simulink model "newStateflow"  (R2018a)
settings: Solver=VariableStepAuto  StartTime=0.0  StopTime=inf  RelTol=1e-3
settings Model: Creator=alex  LastModifiedBy=rohan

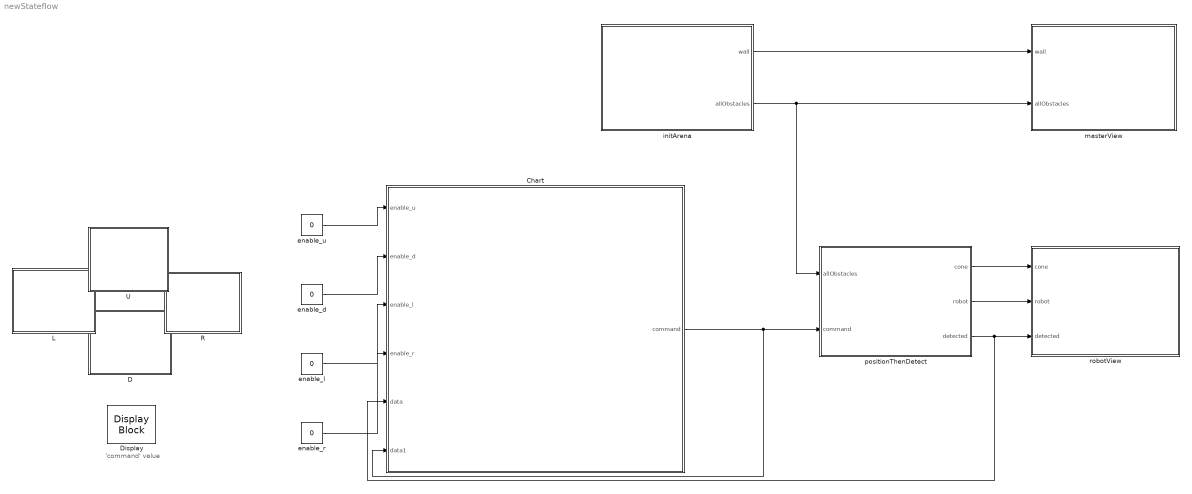
== system newStateflow ==
  note: 'command' value
  Chart : Stateflow chart  TreatAsAtomicUnit=on
  D : Subsystem  DialogController=hmiCreateDDGDialog  IsWebBlock=on  mask(MWDashboardBlock){webBlockId=1a5e94ef-030e-49cd-b944-b929b04abc70, webBlockType=pushbutton, ShowInLibBrwoser=on, ShowInitialText=on, HMISrcModelName=noCollision}
      mask prompts: webBlockId "WebBlock Id"; webBlockType "WebBlock Type"; HMISrcModelName "Source Model"
      mask help: SimulinkHMI:dialogs:PushButtonDialogDesc
      mask Help: helpview([docroot '/mapfiles/simulink.map'], 'hmi_push_button')
      mask Display:
      | model = bdroot(gcb);
      | if strcmp(get_param(model,'BlockDiagramType'), 'library')
      |     image([(matlabroot) '/toolbox/simulink/hmi/icons/PushButton.png']);
      | end
  Display : DisplayBlock  WebBlockId=14  LabelPosition=Hide
  "L " : Subsystem  DialogController=hmiCreateDDGDialog  IsWebBlock=on  mask(MWDashboardBlock){webBlockId=f6d6ee6b-2047-45ee-ab2e-570b521bf019, webBlockType=pushbutton, ShowInLibBrwoser=on, ShowInitialText=on, HMISrcModelName=noCollision}
      mask prompts: webBlockId "WebBlock Id"; webBlockType "WebBlock Type"; HMISrcModelName "Source Model"
      mask help: SimulinkHMI:dialogs:PushButtonDialogDesc
      mask Help: helpview([docroot '/mapfiles/simulink.map'], 'hmi_push_button')
      mask Display:
      | model = bdroot(gcb);
      | if strcmp(get_param(model,'BlockDiagramType'), 'library')
      |     image([(matlabroot) '/toolbox/simulink/hmi/icons/PushButton.png']);
      | end
  R : Subsystem  DialogController=hmiCreateDDGDialog  IsWebBlock=on  mask(MWDashboardBlock){webBlockId=5b3cd59d-fae2-469c-adcb-5a1af564bf62, webBlockType=pushbutton, ShowInLibBrwoser=on, ShowInitialText=on, HMISrcModelName=noCollision}
      mask prompts: webBlockId "WebBlock Id"; webBlockType "WebBlock Type"; HMISrcModelName "Source Model"
      mask help: SimulinkHMI:dialogs:PushButtonDialogDesc
      mask Help: helpview([docroot '/mapfiles/simulink.map'], 'hmi_push_button')
      mask Display:
      | model = bdroot(gcb);
      | if strcmp(get_param(model,'BlockDiagramType'), 'library')
      |     image([(matlabroot) '/toolbox/simulink/hmi/icons/PushButton.png']);
      | end
  U : Subsystem  DialogController=hmiCreateDDGDialog  IsWebBlock=on  mask(MWDashboardBlock){webBlockId=418d2ee9-92ed-471b-995b-1589f387356b, webBlockType=pushbutton, ShowInLibBrwoser=on, ShowInitialText=on, HMISrcModelName=noCollision}
      mask prompts: webBlockId "WebBlock Id"; webBlockType "WebBlock Type"; HMISrcModelName "Source Model"
      mask help: SimulinkHMI:dialogs:PushButtonDialogDesc
      mask Help: helpview([docroot '/mapfiles/simulink.map'], 'hmi_push_button')
      mask Display:
      | model = bdroot(gcb);
      | if strcmp(get_param(model,'BlockDiagramType'), 'library')
      |     image([(matlabroot) '/toolbox/simulink/hmi/icons/PushButton.png']);
      | end
  "enable_d " : Constant  Value=0
  "enable_l " : Constant  Value=0
  "enable_r " : Constant  Value=0
  "enable_u " : Constant  Value=0
  initArena : MATLAB Function  TreatAsAtomicUnit=on
  masterView : MATLAB Function  TreatAsAtomicUnit=on
  positionThenDetect : MATLAB Function  TreatAsAtomicUnit=on
  robotView : MATLAB Function  TreatAsAtomicUnit=on
  wires:
  "enable_u "/1 -> Chart/1(enable_u)
  "enable_d "/1 -> Chart/2(enable_d)
  "enable_l "/1 -> Chart/3(enable_l)
  "enable_r "/1 -> Chart/4(enable_r)
  initArena/1(wall) -> masterView/1(wall)
  initArena/2(allObstacles) -> masterView/2(allObstacles), positionThenDetect/1(allObstacles)
  Chart/1(command) -> Chart/6(data1), positionThenDetect/2(command)
  positionThenDetect/1(cone) -> robotView/1(cone)
  positionThenDetect/2(robot) -> robotView/2(robot)
  positionThenDetect/3(detected) -> Chart/5(data), robotView/3(detected)

== system newStateflow/D ==

== system newStateflow/L  ==

== system newStateflow/R ==

== system newStateflow/U ==

== matlab function newStateflow/initArena ==
  data: wall output; allObstacles output
function [wall, allObstacles] = initArena
    % Clear plot
    clf('reset')
    
    % Parameters 
    xwall = 5756;
    ywall = 3691;
    distance_from_wall = 300;
    
    % Generate field wall 
    wall = generateRectangle(xwall,ywall);

    % Generate virtual limit 
    limit = generateRectangle(xwall-2*distance_from_wall,ywall-2*distance_from_wall);
    limit(:,1) = limit(:,1) + distance_from_wall;
    limit(:,2) = limit(:,2) + distance_from_wall;
    
    % Generate 3 obstacles at semi-random locations 
    size1 = 300;
    size2 = 400;
    size3 = 500; 
    xobst_init = [0,0,0]; yobst_init = [0,0,0];
    for i = 1:3
        xobst_init(i) = randi([size3,xwall-size3]);
        yobst_init(i) = randi([size3,ywall-size3]);
    end
    obstacle1 = generateRectangle(size1, size1);
    obstacle1(:,1) = obstacle1(:,1) + xobst_init(1);
    obstacle1(:,2) = obstacle1(:,2) + yobst_init(1);

    obstacle2 = generateRectangle(size2, size2);
    obstacle2(:,1) = obstacle2(:,1) + xobst_init(2);
    obstacle2(:,2) = obstacle2(:,2) + yobst_init(2);
    
    obstacle3 = generateRectangle(size3, size3);
    obstacle3(:,1) = obstacle3(:,1) + xobst_init(3);
    obstacle3(:,2) = obstacle3(:,2) + yobst_init(3);
    
    % Concatinate all objects into one matrix of x, y, z coordinates
    allObstacles = vertcat(limit, obstacle1, obstacle2, obstacle3);
end

== matlab function newStateflow/positionThenDetect ==
  data: allObstacles input; cone output; command input; robot output; detected output
function [cone, robot, detected] = positionThenDetect(allObstacles, command)
    persistent xpos ypos
    if isempty(xpos)
        xpos = 2000;
        ypos = 2000;
    end
    
    % Base vision cone 
    line1 = [0,150,0; 300,450,0;];
    line2 = [0,150,0; -300,450,0;];
    line3 = [-300,450,0; 300,450,0;];
    base_cone = vertcat(line1, line2, line3);
    
    % Base robot 
    xbase_robot = [0, -100, -100, +100, 100, 0];
    ybase_robot = [150, 50, -150, -150, 50, 150];
    
    % Translate base cone and base robot based on x and y position
    if command == 1
        ypos = ypos + 500;
    elseif command == 2
        ypos = ypos - 500;
    elseif command == 3
        xpos = xpos - 500;
    elseif command == 4
        xpos = xpos + 500;
    end
    % for rotation: come up with a set roation dependent on var and
    %  then make other rotation negative
    % for facing opposite direction: turn 180
    % could do eight cases 

    cone = base_cone;
    cone(:,1) = base_cone(:,1) + xpos;
    cone(:,2) = base_cone(:,2) + ypos;
    cone(:,3) = base_cone(:,3);

    xrobot = xbase_robot + xpos;
    yrobot = ybase_robot + ypos;
    % should concat robot beforehand, like with cone
    robot = fliplr(rot90(vertcat(xrobot,yrobot),3));
    
    %put rotation here--make function in different file

    % Check if obstacle is in vision cone 
    detected = detectObject(allObstacles, cone); 
end

== stateflow chart newStateflow/Chart ==
  state up3
    entry: command = 1
  state down3
    entry: command = 2
  state up2
    entry: command=1
  state left2
    entry: command=3
  state right2
    entry: command=4
  state left3
    entry: command = 3
  state up4
    entry: command = 1
  state down4
    entry: command = 2
  state right4
    entry: command = 4
  state detected_down
    entry: command = 0
  state detected_right
    entry: command = 0
  state detected_left
    entry: command = 0
  state no_input
    entry: command = 0
  state detected_up
    entry: command = 0
  state up
    entry: command = 1
  state down
    entry: command = 2
  state left
    entry: command = 3
  state right
    entry: command = 4
  state down1
    entry:command = 2
  state left1
    entry: command = 3
  state right_1
    entry: command = 4
  detected_down -> up2 [order 2] : [enable_u==1]
  up2 -> detected_down : [enable_u==0]
  detected_down -> left2 [order 4] : [enable_l==1]
  left2 -> detected_down : [enable_l==0]
  right2 -> detected_down : [enable_r==0]
  detected_down -> right2 [order 3] : [enable_r==1]
  detected_right -> up3 [order 3] : [enable_u == 1]
  up3 -> detected_right : [enable_u == 0]
  detected_right -> down3 [order 4] : [enable_d == 1]
  down3 -> detected_right : [enable_d == 0]
  detected_right -> left3 [order 2] : [enable_l == 0]
  left3 -> detected_right : [enable_l == 1]
  detected_left -> up4 [order 3] : [enable_u == 1]
  up4 -> detected_left : [enable_u == 0]
  detected_left -> down4 [order 4] : [enable_d == 1]
  down4 -> detected_left : [enable_d == 0]
  detected_left -> right4 [order 1] : [enable_l == 0]
  detected_up -> no_input [order 3] : [data == 0]
  right4 -> detected_left : [enable_l == 1]
  detected_right -> no_input [order 1] : [data == 0]
  no_input -> detected_right [order 11] : [data == 1]
  no_input -> detected_right [order 12] : [data1 == 4]
  detected_down -> no_input [order 1] : [data == 0]
  no_input -> detected_down [order 9] : [data == 1]
  no_input -> detected_down [order 10] : [data1 == 2]
  (default) -> no_input
  no_input -> detected_up [order 7] : [data==1]
  detected_left -> no_input [order 2] : [data == 0]
  no_input -> detected_left [order 2] : [data == 1]
  no_input -> detected_left [order 3] : [data1 == 3]
  no_input -> detected_up [order 8] : [data1 == 1]
  no_input -> up [order 6] : [enable_u == 1]
  up -> no_input : [enable_u == 0]
  no_input -> down [order 5] : [enable_d ==1]
  down -> no_input : [enable_d == 0]
  no_input -> left [order 4] : [enable_l == 1]
  left -> no_input : [enable_l == 0]
  no_input -> right [order 1] : [enable_r == 1]
  right -> no_input : [enable_r == 0]
  down1 -> detected_up : [enable_d == 0]
  right_1 -> detected_up [order 2] : [enable_r == 0]
  right_1 -> detected_up [order 1] : [enable_r == 1]
  detected_up -> down1 [order 1] : [enable_d ==1]
  detected_up -> left1 [order 2] : [enable_l == 1]
  left1 -> detected_up : [enable_l == 0]
  data: enable_u input; enable_d input; enable_l input; enable_r input; command output; data input; data1 input

== matlab function newStateflow/masterView ==
  data: wall input; allObstacles input
function masterView(wall, allObstacles)
    % Visualize data 
    hold on
    grid on
    grid minor
    xlim([-800 6600])
    ylim([-700 4400])
    plot(wall(:,1), wall(:,2), 'ks-');
    plot(allObstacles(:,1), allObstacles(:,2), 'bs');
    drawnow
end

== matlab function newStateflow/robotView ==
  data: cone input; robot input; detected input
function robotView(cone, robot, detected) 
    % persistent variables are kept local to the function each time it is
    % called 
    persistent coneFig botFig
    
    % coneFig and botFig are initialized as empty, so we can use that to
    % set up a 'run once' part of the funciton that only happens the first
    % time it gets called 
    if isempty(coneFig)
        coneFig = plot(cone(:,1), cone(:,2), 'k.-'); 
        botFig = plot(robot(:,1), robot(:,2), 'k.-'); 
        set([coneFig botFig],'LineWidth', 5)  
        hold off % old objects will be removed 
    end
    
    % need to update the color of the cone if an object is detected 
    if detected 
        coneFig.Color = 'red'; 
    else
        coneFig.Color = 'black';
    end
    
    coneFig.XData = cone(:,1);
    coneFig.YData = cone(:,2);  
    botFig.XData = robot(:,1); 
    botFig.YData = robot(:,2);
    drawnow % update plot without waiting for script to finish 
end
